simulink model "LVLH_error"  (R2021b)
settings: Solver=VariableStepAuto  StartTime=0.0  StopTime=SimTime  RelTol=1e-3
settings Model: Creator=adity  LastModifiedBy=adity

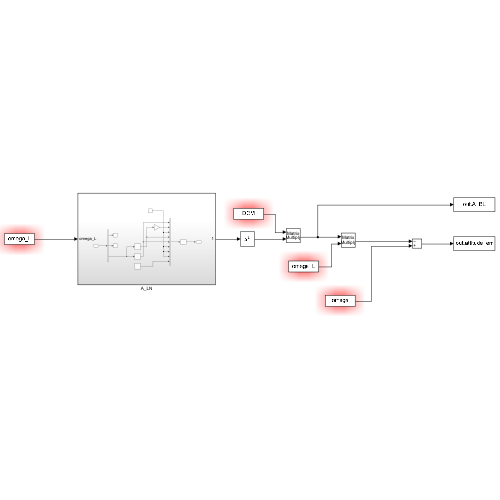
[thumbnail: Simulink's stored preview of the top-level diagram]
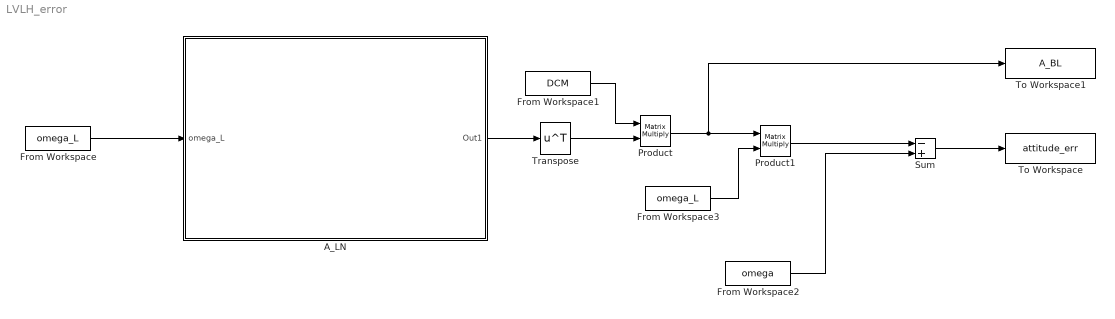
== system LVLH_error ==
  A_LN : Subsystem
  From Workspace : FromWorkspace  VariableName=omega_L
  From Workspace1 : FromWorkspace  VariableName=DCM
  From Workspace2 : FromWorkspace  VariableName=omega
  From Workspace3 : FromWorkspace  VariableName=omega_L
  Product : Product  Multiplication=Matrix(*)
  Product1 : Product  Multiplication=Matrix(*)
  Sum : Sum  Inputs=-+
  To Workspace : ToWorkspace  VariableName=attitude_err  SaveFormat=Timeseries  SampleTime=-1
  To Workspace1 : ToWorkspace  VariableName=A_BL  SaveFormat=Timeseries  SampleTime=-1
  Transpose : Math  Operator=transpose  SaturateOnIntegerOverflow=on
  wires:
  From Workspace/1 -> A_LN/1(omega_L)
  From Workspace2/1 -> Sum/2
  A_LN/1(Out1) -> Transpose/1
  From Workspace1/1 -> Product/1
  Transpose/1 -> Product/2
  Product/1 -> To Workspace1/1, Product1/1
  From Workspace3/1 -> Product1/2
  Product1/1 -> Sum/1
  Sum/1 -> To Workspace/1

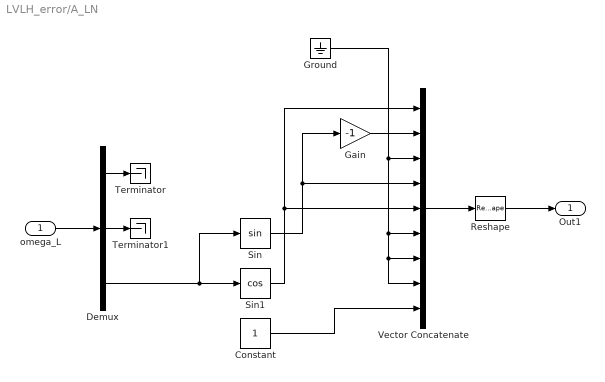
== system LVLH_error/A_LN ==
  omega_L : Inport
  Constant : Constant
  Demux : Demux  Outputs=3
  Gain : Gain  Gain=-1
  Ground : Ground
  Reshape : Reshape  OutputDimensionality=Customize  OutputDimensions=[3,3]
  Sin : Trigonometry
  Sin1 : Trigonometry  Operator=cos
  Terminator : Terminator
  Terminator1 : Terminator
  Vector Concatenate : Concatenate  NumInputs=9
  Out1 : Outport
  wires:
  omega_L/1 -> Demux/1
  Demux/1 -> Terminator/1
  Demux/2 -> Terminator1/1
  Demux/3 -> Sin/1, Sin1/1
  Sin1/1 -> Vector Concatenate/1, Vector Concatenate/5
  Sin/1 -> Gain/1, Vector Concatenate/4
  Ground/1 -> Vector Concatenate/8, Vector Concatenate/7, Vector Concatenate/6, Vector Concatenate/3
  Gain/1 -> Vector Concatenate/2
  Constant/1 -> Vector Concatenate/9
  Vector Concatenate/1 -> Reshape/1
  Reshape/1 -> Out1/1
